simulink model "Radiomaster_joystick_model"  (R2024b)
settings: Solver=VariableStepAuto  StartTime=0.0  StopTime=inf  RelTol=1e-3
libraries: vrlib x1
settings Model: Creator=ada09  LastModifiedBy=ada09

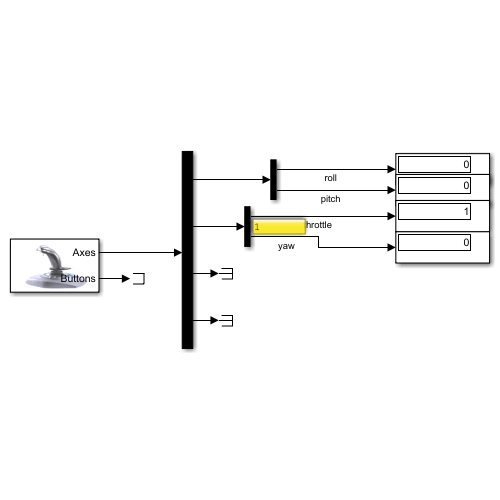
[thumbnail: Simulink's stored preview of the top-level diagram]
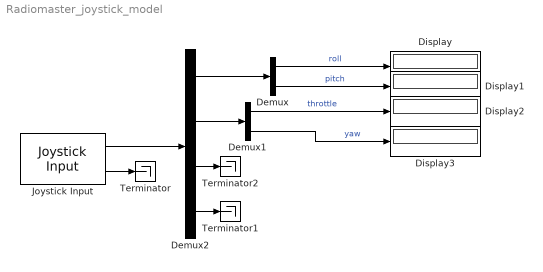
== system Radiomaster_joystick_model ==
  Demux : Demux  Outputs=2
  Demux1 : Demux  Outputs=2
  Demux2 : Demux
  Display{,1..3} (4 alike) : Display
  Joystick Input : vrlib/Joystick Input  joyid=1  adjustports=on  forcefeed=off
  Terminator : Terminator
  Terminator1 : Terminator
  Terminator2 : Terminator
  wires:
  Joystick Input/1 -> Demux2/1
  Joystick Input/2 -> Terminator/1
  Demux2/4 -> Terminator1/1
  Demux2/3 -> Terminator2/1
  Demux2/1 -> Demux/1
  Demux2/2 -> Demux1/1
  Demux/1 -> Display/1  "roll"
  Demux/2 -> Display1/1  "pitch"
  Demux1/1 -> Display2/1  "throttle"
  Demux1/2 -> Display3/1  "yaw"
